simulink model "trig_02b"  (R2022a)
settings: Solver=VariableStepAuto  StartTime=0.0  StopTime=10.0  RelTol=1e-3
settings Model: Creator=FUGAZI  LastModifiedBy=smith

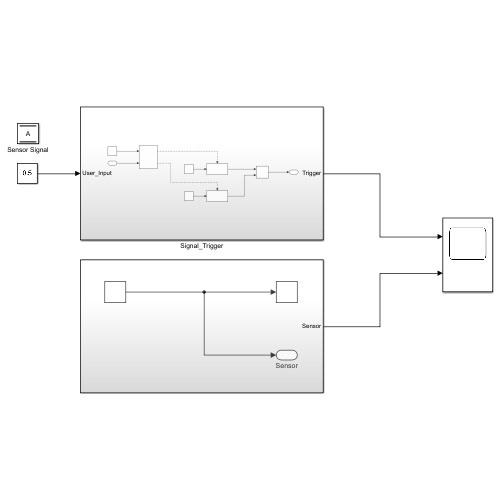
[thumbnail: Simulink's stored preview of the top-level diagram]
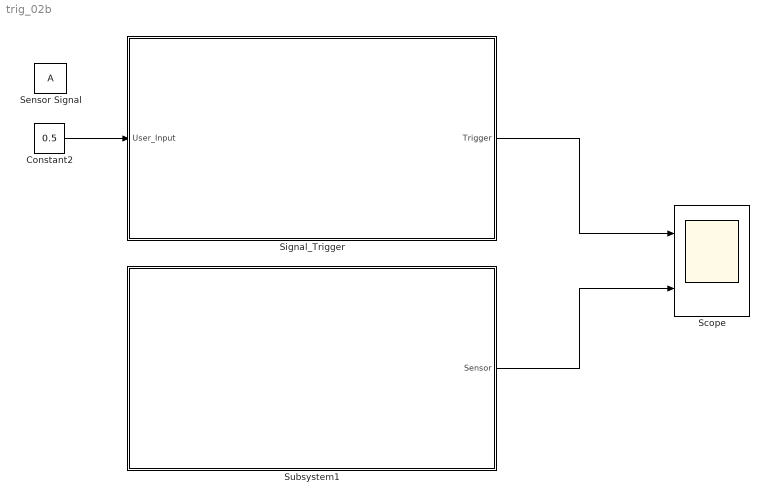
== system trig_02b ==
  Constant2 : Constant  Value=0.5
  Scope : Scope  NumInputPorts=2
  Sensor Signal : DataStoreMemory  WriteAfterWriteMsg=warning  ShowAdditionalParam=off
  Signal_Trigger : Subsystem
  Subsystem1 : Subsystem
  wires:
  Subsystem1/1(Sensor) -> Scope/2
  Signal_Trigger/1(Trigger) -> Scope/1
  Constant2/1 -> Signal_Trigger/1(User_Input)

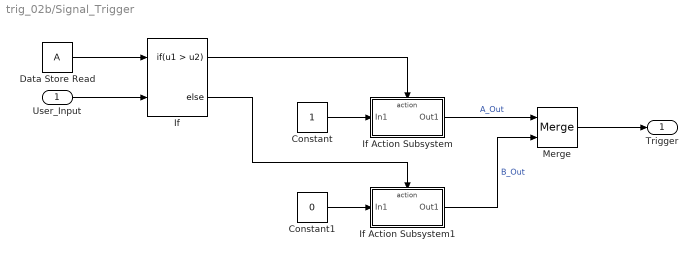
== system trig_02b/Signal_Trigger ==
  User_Input : Inport
  Constant : Constant
  Constant1 : Constant  Value=0
  Data Store Read : DataStoreRead  IndexOptions=Index vector (dialog)  Indices=1  OutputSizes=1
  If : If  NumInputs=2  IfExpression=u1 > u2
  If Action Subsystem : Subsystem  TreatAsAtomicUnit=on
  If Action Subsystem1 : Subsystem  TreatAsAtomicUnit=on
  Merge : Merge
  Trigger : Outport
  wires:
  Constant1/1 -> If Action Subsystem1/1(In1)
  Data Store Read/1 -> If/1
  If/2 -> If Action Subsystem1/Action
  If Action Subsystem/1(Out1) -> Merge/1  "A_Out"
  Constant/1 -> If Action Subsystem/1(In1)
  Merge/1 -> Trigger/1
  If/1 -> If Action Subsystem/Action
  If Action Subsystem1/1(Out1) -> Merge/2  "B_Out"
  User_Input/1 -> If/2

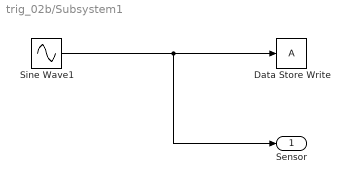
== system trig_02b/Subsystem1 ==
  Data Store Write : DataStoreWrite  IndexOptions=Index vector (dialog)  Indices=1  OutputSizes=1
  Sine Wave1 : Sin  SampleTime=0
  Sensor : Outport
  wires:
  Sine Wave1/1 -> Sensor/1, Data Store Write/1

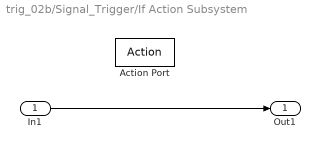
== system trig_02b/Signal_Trigger/If Action Subsystem ==
  In1 : Inport
  Action Port : ActionPort  ActionPortLabel=if(u1 > u2)
  Out1 : Outport
  wires:
  In1/1 -> Out1/1

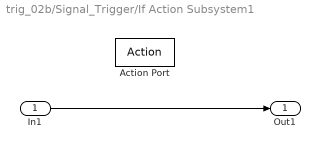
== system trig_02b/Signal_Trigger/If Action Subsystem1 ==
  In1 : Inport
  Action Port : ActionPort  ActionPortLabel=else
  Out1 : Outport
  wires:
  In1/1 -> Out1/1
